simulink model "sTopModel"  (R2021a)
settings: Solver=FixedStepAuto  StartTime=0.0  StopTime=100  FixedStep=Ts  RelTol=1e-3
undefined symbols (not defined in the file or in its folder): dataID, pcktID
libraries: slrealtimeethercatlib x5, simulink x5, slrealtimeutilitieslib x3, slrealtimeiplib x1
settings Model: Creator=Johannes  LastModifiedBy=EGI-Z400
settings SolverCC: ConcurrentTasks=on  AlgebraicLoopSolver=TrustRegion  PositivePriorityOrder=on
settings OptimizationCC: BlockReduction=off  OptimizeBlockIOStorage=off
settings DebuggingCC: TasksWithSamePriorityMsg=none  SFMachineParentedDataDiag=warning
settings HardwareCC: ProdBitPerLong=64  ProdLongLongMode=on  ProdHWDeviceType=Intel->x86-64 (Linux 64)
settings RTWCC: Description=Simulink Real-Time  SystemTargetFile=slrealtime.tlc  TemplateMakefile=slrealtime_default_tmf  RTWVerbose=off  Toolchain=Simulink Real-Time Toolchain  BuildConfiguration=Faster Runs  CodeExecutionProfiling=on  TargetLang=C++

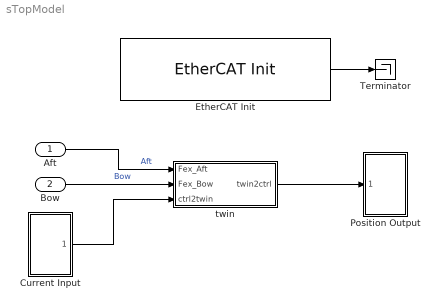
== system sTopModel ==
  Aft : Inport  Interpolate=off
  Bow : Inport  Port=2  Interpolate=off
  Current Input : Subsystem
  EtherCAT Init : slrealtimeethercatlib/EtherCAT Init  Priority=0  config_file=D:\src\sandia\FOSTWIN-Twin\esi\FOSTWIN_Secondary1.xml  device_id=0  pci_bus=0  pci_slot=0  pci_function=0  portnum=1  initstate=2  dctuning=2  enaDebug=0  enaDC=on  errLink=off  masterDbg=off  stateChgDbg=off  baseClock=off  masterCfg=off  logFile='c:\dbglog.txt'  sample_time=0.001000  DCMode=0
      settings: SourceProductBaseCode=XP
  Position Output : Subsystem
  Terminator : Terminator
  twin : Subsystem  Variant=on  VariantControlMode=label  LabelModeActiveChoice=systemID
  wires:
  EtherCAT Init/1 -> Terminator/1
  twin/1(twin2ctrl) -> Position Output/1(twin2ctrl)
  Bow/1 -> twin/2(Fex_Bow)  "Bow"
  Aft/1 -> twin/1(Fex_Aft)  "Aft"
  Current Input/1(ctrl2twin) -> twin/3(ctrl2twin)

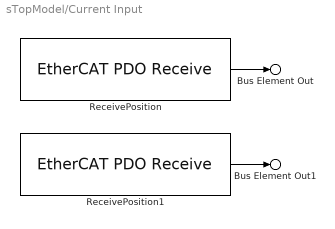
== system sTopModel/Current Input ==
  ReceivePosition : slrealtimeethercatlib/EtherCAT PDO Receive  Priority=2  sig_name=Box 1 (EL6695-0002).IO Inputs.P2S01  sig_offset=328  sig_type=double  type_size=64  sig_dim=1  device_id=0  sample_time=0.001000
      settings: SourceProductBaseCode=XP
  ReceivePosition1 : slrealtimeethercatlib/EtherCAT PDO Receive  Priority=2  sig_name=Box 1 (EL6695-0002).IO Inputs.P2S02  sig_offset=392  sig_type=double  type_size=64  sig_dim=1  device_id=0  sample_time=0.001000
      settings: SourceProductBaseCode=XP
  Bus Element Out : Outport  PortName=ctrl2twin  Element=Cur_Bow
  Bus Element Out1 : Outport  PortName=ctrl2twin  Element=Cur_Aft
  wires:
  ReceivePosition1/1 -> Bus Element Out1/1
  ReceivePosition/1 -> Bus Element Out/1

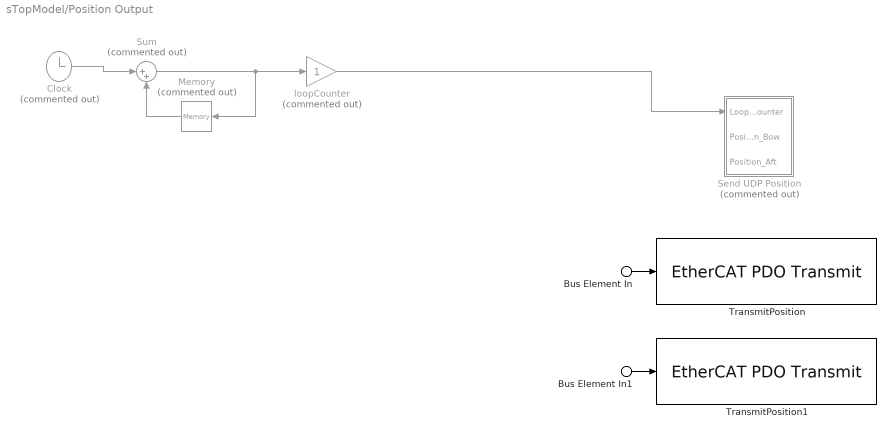
== system sTopModel/Position Output ==
  Bus Element In : Inport  PortName=twin2ctrl  Element=Pos_Bow
  Bus Element In1 : Inport  PortName=twin2ctrl  Element=Pos_Aft
  Clock : Clock  Commented=on
  Memory : Memory  Commented=on
  Send UDP Position : Subsystem  Commented=on
  Sum : Sum  Commented=on  Inputs=|++  OutDataTypeStr=uint32
  TransmitPosition : slrealtimeethercatlib/EtherCAT PDO Transmit  Priority=3  sig_name=Box 1 (EL6695-0002).IO Outputs.S2P01  sig_offset=312  sig_type=double  type_size=64  sig_dim=1  device_id=0  sample_time=0.001000
      settings: SourceProductBaseCode=XP
  TransmitPosition1 : slrealtimeethercatlib/EtherCAT PDO Transmit  Priority=3  sig_name=Box 1 (EL6695-0002).IO Outputs.S2P02  sig_offset=376  sig_type=double  type_size=64  sig_dim=1  device_id=0  sample_time=0.001000
      settings: SourceProductBaseCode=XP
  loopCounter : Gain  Commented=on  ParamDataTypeStr=uint32  OutDataTypeStr=uint32
  wires:
  Memory/1 -> Sum/2
  Clock/1 -> Sum/1
  Sum/1 -> loopCounter/1, Memory/1
  loopCounter/1 -> Send UDP Position/1(LoopCounter)
  Bus Element In1/1 -> TransmitPosition1/1
  Bus Element In/1 -> TransmitPosition/1

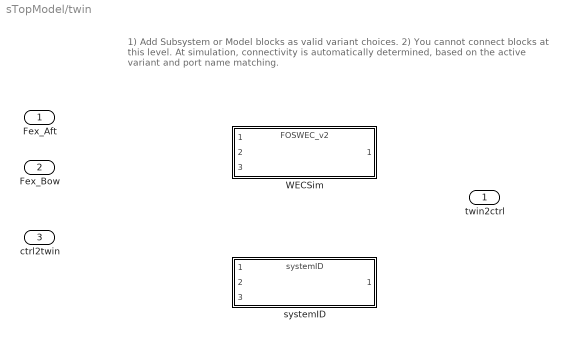
== system sTopModel/twin ==
  note: 1) Add Subsystem or Model blocks as valid variant choices.
      | 2) You cannot connect blocks at this level. At simulation, connectivity is automatically
      | determined, based on the active variant and port name matching.
  Fex_Aft : Inport
  Fex_Bow : Inport  Port=2
  ctrl2twin : Inport  Port=3
  WECSim : ModelReference  ModelNameDialog=FOSWEC_v2.slx  SimulationMode=Normal  VariantControl=WECSim  ModelReferenceVersion=3.288
  systemID : ModelReference  ModelNameDialog=systemID.slx  SimulationMode=Normal  VariantControl=systemID  ModelReferenceVersion=1.83
  twin2ctrl : Outport

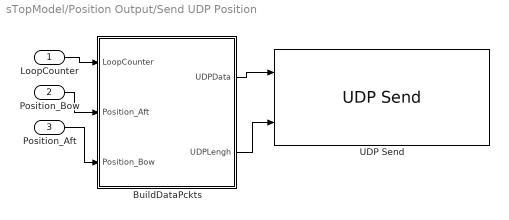
== system sTopModel/Position Output/Send UDP Position ==
  LoopCounter : Inport
  Position_Bow : Inport  Port=2
  Position_Aft : Inport  Port=3
  BuildDataPckts : Subsystem
  UDP Send : slrealtimeiplib/UDP Send  useHostTargetConn=on  ipAddress=10.10.10.15  localPort=iotLocalDataPort  toAddress=iotIPaddr  toPort=iotRemoteDataPort  sampleTime=Ts
      settings: SourceProductBaseCode=XP
  wires:
  Position_Bow/1 -> BuildDataPckts/2(Position_Aft)
  BuildDataPckts/1(UDPData) -> UDP Send/1
  BuildDataPckts/2(UDPLengh) -> UDP Send/2
  LoopCounter/1 -> BuildDataPckts/1(LoopCounter)
  Position_Aft/1 -> BuildDataPckts/3(Position_Bow)

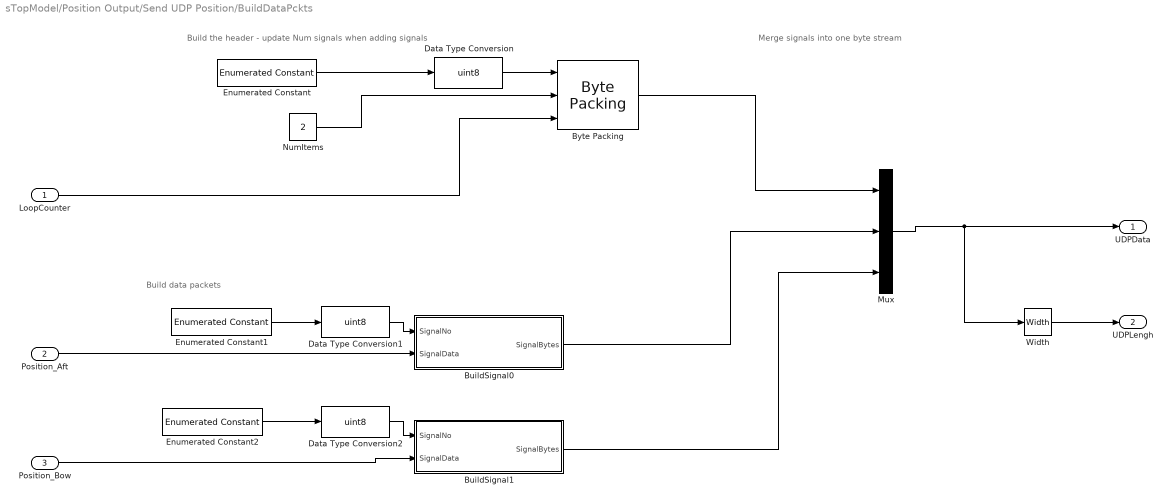
== system sTopModel/Position Output/Send UDP Position/BuildDataPckts ==
  note: Merge signals into one byte stream
  note: Build data packets
  note: Build the header - update Num signals when adding signals
  LoopCounter : Inport
  Position_Aft : Inport  Port=2  OutDataTypeStr=single
  Position_Bow : Inport  Port=3  OutDataTypeStr=single
  BuildSignal0 : Subsystem
  BuildSignal1 : Subsystem
  "Byte Packing " : slrealtimeutilitieslib/Byte Packing  MaskPackedDataType=uint8  MaskUnpackedDataTypes={'uint8','uint8','uint32'}  MaskAlignment=1
  Data Type Conversion : DataTypeConversion  OutDataTypeStr=uint8
  Data Type Conversion1 : DataTypeConversion  OutDataTypeStr=uint8
  Data Type Conversion2 : DataTypeConversion  OutDataTypeStr=uint8
  Enumerated Constant : simulink/Sources/Enumerated Constant  OutDataTypeStr=Enum: pcktID  Value=pcktID.header  SampleTime=inf
  Enumerated Constant1 : simulink/Sources/Enumerated Constant  OutDataTypeStr=Enum: dataID  Value=dataID.position_aft  SampleTime=inf
  Enumerated Constant2 : simulink/Sources/Enumerated Constant  OutDataTypeStr=Enum: dataID  Value=dataID.position_bow  SampleTime=inf
  Mux : Mux  Inputs=3
  NumItems : Constant  Value=2  OutDataTypeStr=uint8
  Width : Width
  UDPData : Outport
  UDPLengh : Outport  Port=2
  wires:
  Width/1 -> UDPLengh/1
  Position_Aft/1 -> BuildSignal0/2(SignalData)
  "Byte Packing "/1 -> Mux/1
  BuildSignal0/1(SignalBytes) -> Mux/2
  BuildSignal1/1(SignalBytes) -> Mux/3
  Mux/1 -> Width/1, UDPData/1
  Data Type Conversion/1 -> "Byte Packing "/1
  Enumerated Constant/1 -> Data Type Conversion/1
  NumItems/1 -> "Byte Packing "/2
  LoopCounter/1 -> "Byte Packing "/3
  Position_Bow/1 -> BuildSignal1/2(SignalData)
  Data Type Conversion1/1 -> BuildSignal0/1(SignalNo)
  Data Type Conversion2/1 -> BuildSignal1/1(SignalNo)
  Enumerated Constant1/1 -> Data Type Conversion1/1
  Enumerated Constant2/1 -> Data Type Conversion2/1

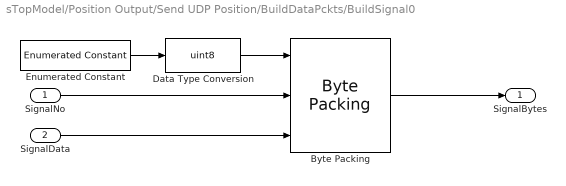
== system sTopModel/Position Output/Send UDP Position/BuildDataPckts/BuildSignal0 ==
  SignalNo : Inport
  SignalData : Inport  Port=2
  "Byte Packing " : slrealtimeutilitieslib/Byte Packing  MaskPackedDataType=uint8  MaskUnpackedDataTypes={'uint8','uint8','single'}  MaskAlignment=1
  Data Type Conversion : DataTypeConversion  OutDataTypeStr=uint8
  Enumerated Constant : simulink/Sources/Enumerated Constant  OutDataTypeStr=Enum: pcktID  Value=pcktID.data  SampleTime=inf
  SignalBytes : Outport
  wires:
  SignalNo/1 -> "Byte Packing "/2
  SignalData/1 -> "Byte Packing "/3
  "Byte Packing "/1 -> SignalBytes/1
  Enumerated Constant/1 -> Data Type Conversion/1
  Data Type Conversion/1 -> "Byte Packing "/1

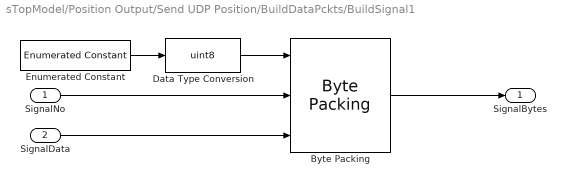
== system sTopModel/Position Output/Send UDP Position/BuildDataPckts/BuildSignal1 ==
  SignalNo : Inport
  SignalData : Inport  Port=2
  "Byte Packing " : slrealtimeutilitieslib/Byte Packing  MaskPackedDataType=uint8  MaskUnpackedDataTypes={'uint8','uint8','single'}  MaskAlignment=1
  Data Type Conversion : DataTypeConversion  OutDataTypeStr=uint8
  Enumerated Constant : simulink/Sources/Enumerated Constant  OutDataTypeStr=Enum: pcktID  Value=pcktID.data  SampleTime=inf
  SignalBytes : Outport
  wires:
  Data Type Conversion/1 -> "Byte Packing "/1
  Enumerated Constant/1 -> Data Type Conversion/1
  "Byte Packing "/1 -> SignalBytes/1
  SignalData/1 -> "Byte Packing "/3
  SignalNo/1 -> "Byte Packing "/2
